simulink model "Systemidentifikation"  (R2023b)
settings: Solver=ode5  StartTime=0.0  StopTime=25  MaxStep=1  RelTol=1e-3  AbsTol=1e-3
InitFcn:
  | if exist('stepFinalValue', 'var')
  |     disp('stepFinalValue exists!');
  | else
  |     stepFinalValue = 1;
  | end
undefined symbols (not defined in the file or in its folder): getservername
libraries: simulink x6
settings Model: Creator=mkottman  LastModifiedBy=Alex
settings SolverCC: AutoScaleAbsTol=off  AlgebraicLoopSolver=TrustRegion
settings DataIOCC: SaveFormat=Array  SignalLoggingSaveFormat=ModelDataLogs  SaveOutput=off  SaveTime=off  ReturnWorkspaceOutputs=off
settings OptimizationCC: BooleanDataType=off  ExpressionDepthLimit=2147483647  InitFltsAndDblsToZero=on  LifeSpan=inf
settings DebuggingCC: SaveWithParameterizedLinksMsg=none  UnderspecifiedInitializationDetection=Classic  MergeDetectMultiDrivingBlocksExec=none  SignalResolutionControl=TryResolveAllWithWarning  MultiTaskDSMMsg=warning  MultiTaskCondExecSysMsg=none  FcnCallInpInsideContextMsg=warning  UnconnectedInputMsg=warning  UnconnectedOutputMsg=warning  UnconnectedLineMsg=warning  StateNameClashWarn=warning  SFUnexpectedBacktrackingDiag=warning  SFNoUnconditionalDefaultTransitionDiag=warning  SFExecutionAtInitializationDiag=none  ArithmeticOperatorsInVariantConditions=warning
settings HardwareCC: ProdBitPerPointer=32  ProdBitPerSizeT=32  ProdBitPerPtrDiffT=32  ProdLargestAtomicFloat=None  ProdIntDivRoundTo=Undefined  ProdEndianess=Unspecified  ProdWordSize=32  ProdHWDeviceType=32-bit Generic  TargetUnknown=on
settings ModelReferenceCC: EnableRefExpFcnMdlSchedulingChecks=on  PropagateSignalLabelsOutOfModel=off
settings SFSimCC: SimUseLocalCustomCode=off  CustomCodeUndefinedFunction=UseInterfaceOnly
settings RTWCC: TemplateMakefile=grt_vc.tmf  RTWUseLocalCustomCode=off
settings CodeAppCC: StateflowObjectComments=on
settings GRTTargetCC: TargetFcnLib=ansi_tfl_tmw.mat  TargetLangStandard=C89/C90 (ANSI)  CombineOutputUpdateFcns=off  GRTInterface=on
settings ConfigComp: CovMetricSettings=dw  CovSaveCumulativeToWorkspaceVar=on  CovSaveSingleToWorkspaceVar=on  CovExternalEMLEnable=off

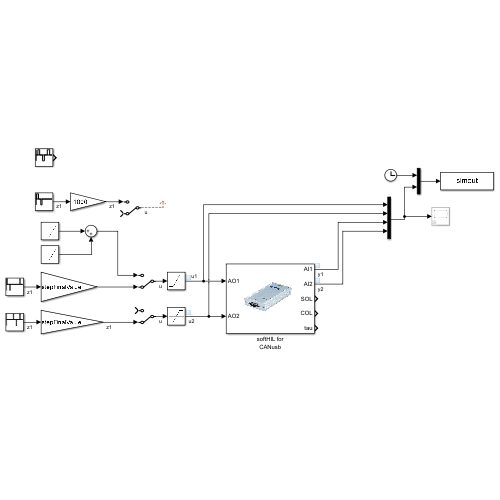
[thumbnail: Simulink's stored preview of the top-level diagram]
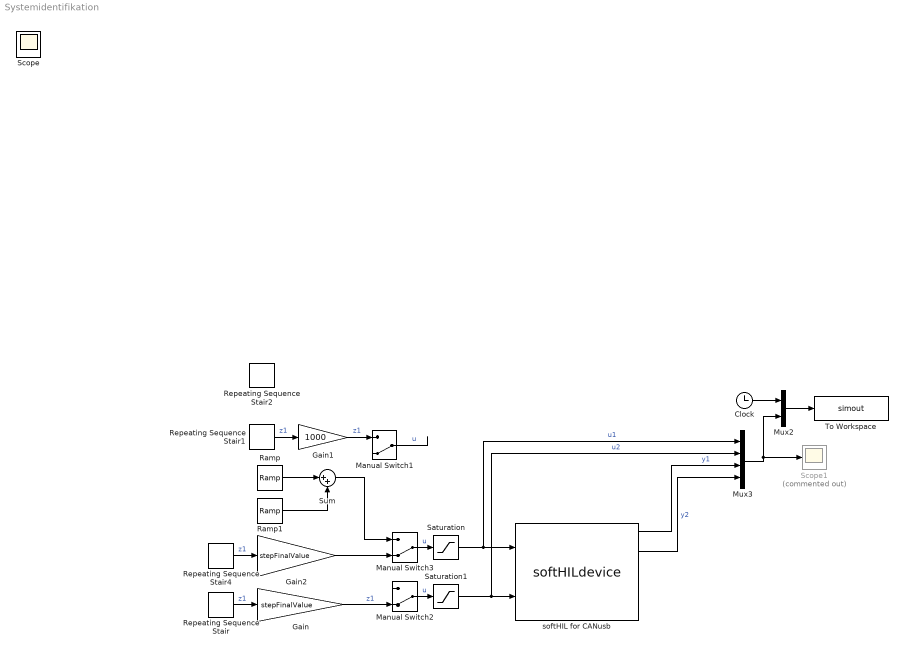
== system Systemidentifikation ==
  Clock : Clock
  Gain : Gain  Gain=stepFinalValue
  Gain1 : Gain  Gain=1000
  Gain2 : Gain  Gain=stepFinalValue
  Manual Switch1 : ManualSwitch  CurrentSetting=0
  Manual Switch2 : ManualSwitch  CurrentSetting=0
  Manual Switch3 : ManualSwitch  CurrentSetting=0
  Mux2 : Mux  Inputs=2
  Mux3 : Mux
  Ramp : simulink/Sources/Ramp  slope=100  start=1  InitialOutput=0
  Ramp1 : simulink/Sources/Ramp  slope=-200  start=8  InitialOutput=0
  Repeating Sequence Stair : simulink/Sources/Repeating Sequence Stair  OutValues=[0 0 0 0 0 0 0 0 0 0 0 0 0 0 0 0 0 0 0 0 0 0 1 0 0 0 0 0 0 0 0 -1 0 0 0 0 0 0 0 0 0 0 1 1 0 0 0 0 0 0 0 0].'  tsamp=0.5  OutMin=[]  OutMax=[]  OutDataTypeStr=double  OutputDataTypeScalingMode=double  OutDataType=fixdt(0,8)  ConRadixGroup=Best Precision: Vector-wise  OutScaling=2^-12
      settings: LibrarySourceBlock=|
      | hdlsllib/Sources/Repeating
      | Sequence
      | Stair
  Repeating Sequence Stair1 : simulink/Sources/Repeating Sequence Stair  OutValues=[0 1 1 0 0 0 -1 -1 0 0 0 0 0 0 0 0 0 0 0 0 0].'  tsamp=1  OutMin=[]  OutMax=[]  OutDataTypeStr=double  OutputDataTypeScalingMode=double  OutDataType=fixdt(0,8)  ConRadixGroup=Best Precision: Vector-wise  OutScaling=2^-12
      settings: LibrarySourceBlock=|
      | hdlsllib/Sources/Repeating
      | Sequence
      | Stair
  Repeating Sequence Stair2 : simulink/Sources/Repeating Sequence Stair  OutValues=[0 0 1 1 0 0 0 -1 -1 0 0 0 1 1 0 0 0].'  tsamp=1  OutMin=[]  OutMax=[]  OutDataTypeStr=double  OutputDataTypeScalingMode=double  OutDataType=fixdt(0,8)  ConRadixGroup=Best Precision: Vector-wise  OutScaling=2^-12
      settings: LibrarySourceBlock=|
      | hdlsllib/Sources/Repeating
      | Sequence
      | Stair
  Repeating Sequence Stair4 : simulink/Sources/Repeating Sequence Stair  OutValues="[0 1 0 0 0 0  0 0 0 0 -1 0 0 0 0 0 0 0 0 0 0 0 0 0 0 0 0 0 0 0 0 0 0 0 0 0 0 0 0 0 0 1 1 0 0 0 0 0 0 0 0  ].'"  tsamp=0.5  OutMin=[]  OutMax=[]  OutDataTypeStr=double  OutputDataTypeScalingMode=double  OutDataType=fixdt(0,8)  ConRadixGroup=Best Precision: Vector-wise  OutScaling=2^-12
      settings: LibrarySourceBlock=|
      | hdlsllib/Sources/Repeating
      | Sequence
      | Stair
  Saturation : Saturate  UpperLimit=3000  LowerLimit=-3000
  Saturation1 : Saturate  UpperLimit=3000  LowerLimit=-3000
  Scope1 : Scope  Commented=on
  Sum : Sum  Inputs=|++
  To Workspace : ToWorkspace  VariableName=simout  SampleTime=0.01
  softHIL for CANusb : S-Function  FunctionName=softHILdevice  Parameters=nAIn, nAOut, nDIn, nDOut, 0, Sampletime, Servername, ServerOL, ClientOL, Delay, 'CANusb'  SFunctionDeploymentMode=off  EnableBusSupport=off  mask(softHIL for the CANusb){nAIn=2, nAOut=2, nDIn=0, nDOut=0, Sampletime=0.01, Servername=getservername, ServerOL=on, ClientOL=on, Delay=on}
      mask prompts: nAIn "Number of Analog In (AI)"; nAOut "Number of Analog Out (AO)"; nDIn "Number of Digital In (DI)"; nDOut "Number of Digital Out (DO)"; Sampletime "Sample Time"; ServerOL "Show Server Overloads Port"; ClientOL "Show Client Overloads Port"; Delay "Show Roundtrip Delay Port"
      mask help: softHIL (soft hardware in the loop) for the CANusb device.
      mask Help:
      | softHIL (soft hardware in the loop) for the CANusb allows to connect to a remote server (over TCP and UDP) which runs the SoftHILServer service to acquire from and deliver data to the device. This version is limited to work for the setup at the Control Engineering Laboratories of the University of Applied Sciences HSR in Rapperswil, CH.
      | 
      | The implementation of the softing CANusb device was only made for the process “Schwungmasse“. If you want to use the device in a different function it’s recommended to use it directly.
      | 
      | <big><b>Ports</b></big>
      | <table border=1><tr><td>Portname</td><td>Description</td><td>Min</td><td>Max</td></tr><tr><td>AO1/A2</td><td>Analog Outputs</td><td>-</td><td>-</td></tr><tr><td>AI1/AI2</td><td>Analog Inputs</td><td>-</td><td>-</td></tr><tr><td>SOL</td><td>Whenever the server is not able to finish the acquisition of the samples at the specified sample time, a server overload occurs and the SOL (Server Overloads) counter will increment by 1.</td><td>0</td><td>2^31</td></tr><tr><td>COL</td><td>Whenever the client is not able to finish its calculations until the next samples arrive, a client overload occurs and the COL (Client Overloads) counter will increment by 1.</td><td>0</td><td>2^31</td></tr><tr><td>tau</td><td>tau specifies the current roundtrip delay. It is a measure of the delay due to the network (protocol stack, switches, etc.)</td><td>0</td><td>-</td></tr></table>
      | <br>
      | <big><b>Parameters</b></big>
      | <table border="1"><tr><td>Parametername</td><td>Description</td><td>Min</td><td>Max</td></tr><tr><td>Number of Analog In (AI)</td><td>A scalar value that specifies the number of analog input channels the I/O board should acquire. Should be 2!</td><td>0</td><td>8</td></tr><tr><td>Number of Analog Out (AO)</td><td>A scalar value that specifies the number of analog output channels the I/O board should write to. Should be 2!</td><td>0</td><td>6</td></tr><tr><td>Number of Digital In (DI)</td><td>A scalar value that specifies the number of digital input channels the I/O board should acquire. Should be 0!</td><td>0</td><td>8</td></tr><tr><td>Number of Digital Out (DO)</td><td>A scalar value that specifies the number of digital output channels the I/O board should set. Should be 0!</td><td>0</td><td>8</td></tr><tr><td>Sample Time</td><td>A scalar value that specifies the sampling rate (in seconds) at which the I/O board acquires data and at which rate the softHIL block sends new output values to the server. The rate has to be a multiple of 1ms.</td><td>0.001</td><td>-</td></tr><tr><td>Servername</td><td>The name or IP address of the server on which the SoftHILServer service is running and the I/O boards are installed. This argument has to be a string. Use 'localhost' if the server runs on the same machine.</td><td>-</td><td>-</td></tr><tr><td>Show Server Overload Port</td><td>Check to see the 'SOL' output port.</td><td>-</td><td>-</td></tr><tr><td>Show Client Overload Port</td><td>Check to see the 'COL' output port.</td><td>-</td><td>-</td></tr><tr><td>Show Roundtrip Delay Port</td><td>Check to see the 'tau' output port.</td><td>-</td><td>-</td></tr></table>
      | <br>
      | <big style="font-weight: bold;">Hints</big><br>
      | <ul>
      | <li>It can happen that Simulink freezes during simulation due to a connection problem with the server. In this case, restart the SoftHILServer service on the server. As soon as the service quits, Simulink will enter a normal error state and stop the simulation. Check the Event Log of the server to get some information about the cause of the problem.</li>
      | <li>When you receive a 'configuration error' and the Simulation does not start, make sure that the number of channels are in the correct range and check the Event Log on the server for further information. Make sure to have the correct InstaCal installed on the server and the boards are properly configured.</li>
      | <li>The server and the client run on Windows, which is not a RealTime operating system. Execution accuracy depends on the available system resources. Do not do anything else with the system during simulations to improve accuracy.</li>
      | <li>Check SOL and COL output ports to make sure the server and the client are able to deliver the required sample time. Some overloads during the start of the simulation are normal. While the simulation is running, these counters should not continuously increase. If this happens, the RealTime condition is hardly violated. Increase the sample time and/or reduce model complexity.</li>
      | <li>The more values are read from and written to the I/O board, the longer the A/D and D/A conversions will take. It is possible that the lower bound of 1ms is not possible any more, even for the simplest model and fastes processors. Check the server overload counter (SOL) to detect this problem.</li>
      | </ul>
      mask Display:
      | image(imread('CANusb.jpg'));
      | 
      | nAIn = str2num(get_param(gcb, 'nAIn'));
      | nDIn = str2num(get_param(gcb, 'nDIn'));
      | nAOut = str2num(get_param(gcb, 'nAOut'));
      | nDOut = str2num(get_param(gcb, 'nDOut'));
      | 
      | offset = 0;
      | for i = 1:nAIn
      |     port_label('output', i + offset, ['AI' num2str(i)]);
      | end
      | offset = offset + nAIn;
      | for i = 1:nDIn
      |     port_label('output', i + offset, ['DI', num2str(i)]);
      | end
      | offset = offset + nDIn;
      | if strcmp(get_param(gcb, 'ServerOL'), 'on')
      |     port_label('output', 1 + offset, 'SOL');
      |     offset = offset + 1;
      | end
      | if strcmp(get_param(gcb, 'ClientOL'), 'on')
      |     port_label('output', 1 + offset, 'COL');
      |     offset = offset + 1;
      | end
      | if strcmp(get_param(gcb, 'Delay'), 'on')
      |     port_label('output', 1 + offset, 'tau');
      |     offset = offset + 1;
      | end
      | 
      | offset = 0;
      | for i = 1:nAOut
      |     port_label('input', i + offset, ['AO' num2str(i)]);
      | end
      | offset = offset + nAOut;
      | for i = 1:nDOut
      |     port_label('input', i + offset, ['DO', num2str(i)]);
      | end
  Scope : Scope
  wires:
  Saturation1/1 -> Mux3/2, softHIL for CANusb/2  "u2"
  Saturation/1 -> Mux3/1, softHIL for CANusb/1  "u1"
  Repeating Sequence Stair/1 -> Gain/1  "z1"
  Gain1/1 -> Manual Switch1/1  "z1"
  Repeating Sequence Stair1/1 -> Gain1/1  "z1"
  Repeating Sequence Stair4/1 -> Gain2/1  "z1"
  Manual Switch1/1 -> ?  "u"
  Gain/1 -> Manual Switch2/2  "z1"
  Clock/1 -> Mux2/1
  Mux3/1 -> Scope1/1, Mux2/2
  Mux2/1 -> To Workspace/1
  softHIL for CANusb/1 -> Mux3/3  "y1"
  softHIL for CANusb/2 -> Mux3/4  "y2"
  Manual Switch2/1 -> Saturation1/1  "u"
  Manual Switch3/1 -> Saturation/1  "u"
  Ramp/1 -> Sum/1
  Gain2/1 -> Manual Switch3/2
  Ramp1/1 -> Sum/2
  Sum/1 -> Manual Switch3/1
